simulink model "case5"  (R2024b)
settings: Solver=FixedStepAuto  StartTime=0  StopTime=1  FixedStep=1e-7  RelTol=1e-3
values from neighbouring files (symbols this model uses):
  SG_D_1_D = 0.01056    [IEEE9_case_parameters.m]    (also in case1_parameters.m; case2_parameters.m; case3_parameters.m; case4_parameters.m)
  SG_D_1_EnableSaturation = 0    [IEEE9_case_parameters.m]    (also in case1_parameters.m; case2_parameters.m; case3_parameters.m; case4_parameters.m)
  SG_D_1_f0 = 60    [IEEE9_case_parameters.m]    (also in case1_parameters.m; case2_parameters.m; case3_parameters.m; case4_parameters.m)
  SG_D_1_H = 7.5    [IEEE9_case_parameters.m]    (also in case1_parameters.m; case2_parameters.m; case3_parameters.m; case4_parameters.m)
  SG_D_1_K_A = 20    [IEEE9_case_parameters.m]    (also in case1_parameters.m; case2_parameters.m; case3_parameters.m; case4_parameters.m)
  SG_D_1_K_E = 1.000000e+1    (= 10)    [IEEE9_case_parameters.m]    (also in case1_parameters.m; case2_parameters.m; case3_parameters.m; case4_parameters.m)
  SG_D_1_K_F = 2.363    [IEEE9_case_parameters.m]    (also in case1_parameters.m; case2_parameters.m; case3_parameters.m; case4_parameters.m)
  SG_D_1_K_s = 0.5    [IEEE9_case_parameters.m]    (also in case1_parameters.m = 5; case2_parameters.m = 5; case3_parameters.m = 5; case4_parameters.m = 5)
  SG_D_1_R_a = 0.001088    [IEEE9_case_parameters.m]    (also in case1_parameters.m; case2_parameters.m; case3_parameters.m; case4_parameters.m)
  SG_D_1_S_A = 1    [IEEE9_case_parameters.m]    (also in case1_parameters.m; case2_parameters.m; case3_parameters.m; case4_parameters.m)
  SG_D_1_S_B = 0.103    [IEEE9_case_parameters.m]    (also in case1_parameters.m; case2_parameters.m; case3_parameters.m; case4_parameters.m)
  SG_D_1_S_N = 10.659857    [IEEE9_case_parameters.m]    (also in case1_parameters.m; case2_parameters.m; case3_parameters.m; case4_parameters.m)
  SG_D_1_SpeedPara = 200    [IEEE9_case_parameters.m]    (also in case1_parameters.m; case2_parameters.m; case3_parameters.m; case4_parameters.m)
  SG_D_1_T_0 = 0.720173    [IEEE9_case_parameters.m]    (also in case1_parameters.m = 0.755522; case2_parameters.m = 0.808931; case3_parameters.m = 0.869402; case4_parameters.m = 0.729316)
  SG_D_1_T_1 = 0.3    [IEEE9_case_parameters.m]    (also in case1_parameters.m; case2_parameters.m; case3_parameters.m; case4_parameters.m)
  SG_D_1_T_2 = 0.05    [IEEE9_case_parameters.m]    (also in case1_parameters.m; case2_parameters.m; case3_parameters.m; case4_parameters.m)
  SG_D_1_T_3 = 0.02    [IEEE9_case_parameters.m]    (also in case1_parameters.m; case2_parameters.m; case3_parameters.m; case4_parameters.m)
  SG_D_1_T_4 = 0.005    [IEEE9_case_parameters.m]    (also in case1_parameters.m; case2_parameters.m; case3_parameters.m; case4_parameters.m)
  SG_D_1_T_A = 0.02    [IEEE9_case_parameters.m]    (also in case1_parameters.m; case2_parameters.m; case3_parameters.m; case4_parameters.m)
  SG_D_1_T_dd = 8.000000e+0    (= 8)    [IEEE9_case_parameters.m]    (also in case1_parameters.m; case2_parameters.m; case3_parameters.m; case4_parameters.m)
  SG_D_1_T_ddd = 0.04    [IEEE9_case_parameters.m]    (also in case1_parameters.m; case2_parameters.m; case3_parameters.m; case4_parameters.m)
  SG_D_1_T_E = 0.314    [IEEE9_case_parameters.m]    (also in case1_parameters.m; case2_parameters.m; case3_parameters.m; case4_parameters.m)
  SG_D_1_T_F = 0.35    [IEEE9_case_parameters.m]    (also in case1_parameters.m; case2_parameters.m; case3_parameters.m; case4_parameters.m)
  SG_D_1_T_qd = 0.8    [IEEE9_case_parameters.m]    (also in case1_parameters.m; case2_parameters.m; case3_parameters.m; case4_parameters.m)
  SG_D_1_T_qdd = 0.02    [IEEE9_case_parameters.m]    (also in case1_parameters.m; case2_parameters.m; case3_parameters.m; case4_parameters.m)
  SG_D_1_T_speed = 0.1    [IEEE9_case_parameters.m]    (also in case1_parameters.m = 200; case2_parameters.m = 200; case3_parameters.m = 200; case4_parameters.m = 200)
  SG_D_1_T_w = 0.5    [IEEE9_case_parameters.m]    (also in case1_parameters.m; case2_parameters.m; case3_parameters.m; case4_parameters.m)
  SG_D_1_V_ref = 1.990276    [IEEE9_case_parameters.m]    (also in case1_parameters.m = 2.042296; case2_parameters.m = 2.051388; case3_parameters.m = 2.089584; case4_parameters.m = 2.01845)
  SG_D_1_w_ref = 376.991118    [IEEE9_case_parameters.m]    (also in case1_parameters.m; case2_parameters.m; case3_parameters.m; case4_parameters.m)
  SG_D_1_wb = 6.000000e+1    (= 60)    [IEEE9_case_parameters.m]    (also in case1_parameters.m; case2_parameters.m; case3_parameters.m; case4_parameters.m)
  SG_D_1_x_d = 1.9    [IEEE9_case_parameters.m]    (also in case1_parameters.m; case2_parameters.m; case3_parameters.m; case4_parameters.m)
  SG_D_1_x_dd = 0.302    [IEEE9_case_parameters.m]    (also in case1_parameters.m; case2_parameters.m; case3_parameters.m; case4_parameters.m)
  SG_D_1_x_ddd = 0.204    [IEEE9_case_parameters.m]    (also in case1_parameters.m; case2_parameters.m; case3_parameters.m; case4_parameters.m)
  SG_D_1_x_l = 0.05    [IEEE9_case_parameters.m]    (also in case1_parameters.m; case2_parameters.m; case3_parameters.m; case4_parameters.m)
  SG_D_1_x_q = 1.3    [IEEE9_case_parameters.m]    (also in case1_parameters.m; case2_parameters.m; case3_parameters.m; case4_parameters.m)
  SG_D_1_x_qd = 0.5    [IEEE9_case_parameters.m]    (also in case1_parameters.m; case2_parameters.m; case3_parameters.m; case4_parameters.m)
  SG_D_1_x_qdd = 0.3    [IEEE9_case_parameters.m]    (also in case1_parameters.m; case2_parameters.m; case3_parameters.m; case4_parameters.m)
  SG_D_2_D = 0.02    [IEEE9_case_parameters.m]    (also in case1_parameters.m; case2_parameters.m; case3_parameters.m; case4_parameters.m)
  SG_D_2_EnableSaturation = 0    [IEEE9_case_parameters.m]    (also in case1_parameters.m; case2_parameters.m; case3_parameters.m; case4_parameters.m)
  SG_D_2_f0 = 60    [IEEE9_case_parameters.m]    (also in case1_parameters.m; case2_parameters.m; case3_parameters.m; case4_parameters.m)
  SG_D_2_H = 8.000000e+0    (= 8)    [IEEE9_case_parameters.m]    (also in case1_parameters.m; case2_parameters.m; case3_parameters.m; case4_parameters.m)
  SG_D_2_K_A = 20    [IEEE9_case_parameters.m]    (also in case1_parameters.m; case2_parameters.m; case3_parameters.m; case4_parameters.m)
  SG_D_2_K_E = 1.000000e+1    (= 10)    [IEEE9_case_parameters.m]    (also in case1_parameters.m; case2_parameters.m; case3_parameters.m; case4_parameters.m)
  SG_D_2_K_F = 2.363    [IEEE9_case_parameters.m]    (also in case1_parameters.m; case2_parameters.m; case3_parameters.m; case4_parameters.m)
  SG_D_2_K_s = 0.5    [IEEE9_case_parameters.m]    (also in case1_parameters.m = 4; case2_parameters.m = 4; case3_parameters.m = 4; case4_parameters.m = 4)
  SG_D_2_R_a = 0.001088    [IEEE9_case_parameters.m]    (also in case1_parameters.m; case2_parameters.m; case3_parameters.m; case4_parameters.m)
  SG_D_2_S_A = 1    [IEEE9_case_parameters.m]    (also in case1_parameters.m; case2_parameters.m; case3_parameters.m; case4_parameters.m)
  SG_D_2_S_B = 0.103    [IEEE9_case_parameters.m]    (also in case1_parameters.m; case2_parameters.m; case3_parameters.m; case4_parameters.m)
  SG_D_2_S_N = 10.659857    [IEEE9_case_parameters.m]    (also in case1_parameters.m; case2_parameters.m; case3_parameters.m; case4_parameters.m)
  SG_D_2_SpeedPara = 200    [IEEE9_case_parameters.m]    (also in case1_parameters.m; case2_parameters.m; case3_parameters.m; case4_parameters.m)
  SG_D_2_T_0 = 1.632913    [IEEE9_case_parameters.m]    (also in case1_parameters.m = 1.632925; case2_parameters.m = 1.632915; case3_parameters.m = 1.632914; case4_parameters.m = 1.632927)
  SG_D_2_T_1 = 0.2    [IEEE9_case_parameters.m]    (also in case1_parameters.m; case2_parameters.m; case3_parameters.m; case4_parameters.m)
  SG_D_2_T_2 = 0.05    [IEEE9_case_parameters.m]    (also in case1_parameters.m; case2_parameters.m; case3_parameters.m; case4_parameters.m)
  SG_D_2_T_3 = 0.02    [IEEE9_case_parameters.m]    (also in case1_parameters.m; case2_parameters.m; case3_parameters.m; case4_parameters.m)
  SG_D_2_T_4 = 0.005    [IEEE9_case_parameters.m]    (also in case1_parameters.m; case2_parameters.m; case3_parameters.m; case4_parameters.m)
  SG_D_2_T_A = 0.02    [IEEE9_case_parameters.m]    (also in case1_parameters.m; case2_parameters.m; case3_parameters.m; case4_parameters.m)
  SG_D_2_T_dd = 7.9    [IEEE9_case_parameters.m]    (also in case1_parameters.m; case2_parameters.m; case3_parameters.m; case4_parameters.m)
  SG_D_2_T_ddd = 0.04    [IEEE9_case_parameters.m]    (also in case1_parameters.m; case2_parameters.m; case3_parameters.m; case4_parameters.m)
  SG_D_2_T_E = 0.314    [IEEE9_case_parameters.m]    (also in case1_parameters.m; case2_parameters.m; case3_parameters.m; case4_parameters.m)
  SG_D_2_T_F = 0.35    [IEEE9_case_parameters.m]    (also in case1_parameters.m; case2_parameters.m; case3_parameters.m; case4_parameters.m)
  SG_D_2_T_qd = 0.8    [IEEE9_case_parameters.m]    (also in case1_parameters.m; case2_parameters.m; case3_parameters.m; case4_parameters.m)
  SG_D_2_T_qdd = 0.015    [IEEE9_case_parameters.m]    (also in case1_parameters.m; case2_parameters.m; case3_parameters.m; case4_parameters.m)
  SG_D_2_T_speed = 0.1    [IEEE9_case_parameters.m]    (also in case1_parameters.m = 150; case2_parameters.m = 150; case3_parameters.m = 150; case4_parameters.m = 150)
  SG_D_2_T_w = 0.35    [IEEE9_case_parameters.m]    (also in case1_parameters.m; case2_parameters.m; case3_parameters.m; case4_parameters.m)
  SG_D_2_V_ref = 2.58547    [IEEE9_case_parameters.m]    (also in case1_parameters.m = 2.597896; case2_parameters.m = 2.587136; case3_parameters.m = 2.586042; case4_parameters.m = 2.599679)
  SG_D_2_w_ref = 376.991118    [IEEE9_case_parameters.m]    (also in case1_parameters.m; case2_parameters.m; case3_parameters.m; case4_parameters.m)
  SG_D_2_wb = 6.000000e+1    (= 60)    [IEEE9_case_parameters.m]    (also in case1_parameters.m; case2_parameters.m; case3_parameters.m; case4_parameters.m)
  SG_D_2_x_d = 1.8    [IEEE9_case_parameters.m]    (also in case1_parameters.m; case2_parameters.m; case3_parameters.m; case4_parameters.m)
  SG_D_2_x_dd = 0.302    [IEEE9_case_parameters.m]    (also in case1_parameters.m; case2_parameters.m; case3_parameters.m; case4_parameters.m)
  SG_D_2_x_ddd = 0.204    [IEEE9_case_parameters.m]    (also in case1_parameters.m; case2_parameters.m; case3_parameters.m; case4_parameters.m)
  SG_D_2_x_l = 0.05    [IEEE9_case_parameters.m]    (also in case1_parameters.m; case2_parameters.m; case3_parameters.m; case4_parameters.m)
  SG_D_2_x_q = 1.25    [IEEE9_case_parameters.m]    (also in case1_parameters.m; case2_parameters.m; case3_parameters.m; case4_parameters.m)
  SG_D_2_x_qd = 0.5    [IEEE9_case_parameters.m]    (also in case1_parameters.m; case2_parameters.m; case3_parameters.m; case4_parameters.m)
  SG_D_2_x_qdd = 0.3    [IEEE9_case_parameters.m]    (also in case1_parameters.m; case2_parameters.m; case3_parameters.m; case4_parameters.m)
  SG_D_3_D = 0.02    [IEEE9_case_parameters.m]    (also in case1_parameters.m; case2_parameters.m; case3_parameters.m; case4_parameters.m)
  SG_D_3_EnableSaturation = 0    [IEEE9_case_parameters.m]    (also in case1_parameters.m; case2_parameters.m; case3_parameters.m; case4_parameters.m)
  SG_D_3_f0 = 60    [IEEE9_case_parameters.m]    (also in case1_parameters.m; case2_parameters.m; case3_parameters.m; case4_parameters.m)
  SG_D_3_H = 7.7    [IEEE9_case_parameters.m]    (also in case1_parameters.m; case2_parameters.m; case3_parameters.m; case4_parameters.m)
  SG_D_3_K_A = 20    [IEEE9_case_parameters.m]    (also in case1_parameters.m; case2_parameters.m; case3_parameters.m; case4_parameters.m)
  SG_D_3_K_E = 1.000000e+1    (= 10)    [IEEE9_case_parameters.m]    (also in case1_parameters.m; case2_parameters.m; case3_parameters.m; case4_parameters.m)
  SG_D_3_K_F = 2.363    [IEEE9_case_parameters.m]    (also in case1_parameters.m; case2_parameters.m; case3_parameters.m; case4_parameters.m)
  SG_D_3_K_s = 0.2    [IEEE9_case_parameters.m]    (also in case1_parameters.m = 2; case2_parameters.m = 2; case3_parameters.m = 2; case4_parameters.m = 2)
  SG_D_3_R_a = 0.001088    [IEEE9_case_parameters.m]    (also in case1_parameters.m; case2_parameters.m; case3_parameters.m; case4_parameters.m)
  SG_D_3_S_A = 1    [IEEE9_case_parameters.m]    (also in case1_parameters.m; case2_parameters.m; case3_parameters.m; case4_parameters.m)
  SG_D_3_S_B = 0.103    [IEEE9_case_parameters.m]    (also in case1_parameters.m; case2_parameters.m; case3_parameters.m; case4_parameters.m)
  SG_D_3_S_N = 10.659857    [IEEE9_case_parameters.m]    (also in case1_parameters.m; case2_parameters.m; case3_parameters.m; case4_parameters.m)
  SG_D_3_SpeedPara = 200    [IEEE9_case_parameters.m]    (also in case1_parameters.m; case2_parameters.m; case3_parameters.m; case4_parameters.m)
  SG_D_3_T_0 = 0.850788    [IEEE9_case_parameters.m]    (also in case1_parameters.m = 0.850786; case2_parameters.m = 0.850787; case3_parameters.m; case4_parameters.m = 0.850786)
  SG_D_3_T_1 = 0.2    [IEEE9_case_parameters.m]    (also in case1_parameters.m; case2_parameters.m; case3_parameters.m; case4_parameters.m)
  SG_D_3_T_2 = 0.05    [IEEE9_case_parameters.m]    (also in case1_parameters.m; case2_parameters.m; case3_parameters.m; case4_parameters.m)
  SG_D_3_T_3 = 0.02    [IEEE9_case_parameters.m]    (also in case1_parameters.m; case2_parameters.m; case3_parameters.m; case4_parameters.m)
  SG_D_3_T_4 = 0.005    [IEEE9_case_parameters.m]    (also in case1_parameters.m; case2_parameters.m; case3_parameters.m; case4_parameters.m)
  SG_D_3_T_A = 0.02    [IEEE9_case_parameters.m]    (also in case1_parameters.m; case2_parameters.m; case3_parameters.m; case4_parameters.m)
  SG_D_3_T_dd = 8.1    [IEEE9_case_parameters.m]    (also in case1_parameters.m; case2_parameters.m; case3_parameters.m; case4_parameters.m)
  SG_D_3_T_ddd = 0.04    [IEEE9_case_parameters.m]    (also in case1_parameters.m; case2_parameters.m; case3_parameters.m; case4_parameters.m)
  SG_D_3_T_E = 0.314    [IEEE9_case_parameters.m]    (also in case1_parameters.m; case2_parameters.m; case3_parameters.m; case4_parameters.m)
  SG_D_3_T_F = 0.35    [IEEE9_case_parameters.m]    (also in case1_parameters.m; case2_parameters.m; case3_parameters.m; case4_parameters.m)
  SG_D_3_T_qd = 0.8    [IEEE9_case_parameters.m]    (also in case1_parameters.m; case2_parameters.m; case3_parameters.m; case4_parameters.m)
  SG_D_3_T_qdd = 0.015    [IEEE9_case_parameters.m]    (also in case1_parameters.m; case2_parameters.m; case3_parameters.m; case4_parameters.m)
  SG_D_3_T_speed = 0.1    [IEEE9_case_parameters.m]    (also in case1_parameters.m = 180; case2_parameters.m = 180; case3_parameters.m = 180; case4_parameters.m = 180)
  SG_D_3_T_w = 0.4    [IEEE9_case_parameters.m]    (also in case1_parameters.m; case2_parameters.m; case3_parameters.m; case4_parameters.m)
  SG_D_3_V_ref = 1.892727    [IEEE9_case_parameters.m]    (also in case1_parameters.m = 1.906439; case2_parameters.m = 1.895535; case3_parameters.m = 1.892105; case4_parameters.m = 1.906598)
  SG_D_3_w_ref = 376.991118    [IEEE9_case_parameters.m]    (also in case1_parameters.m; case2_parameters.m; case3_parameters.m; case4_parameters.m)
  SG_D_3_wb = 6.000000e+1    (= 60)    [IEEE9_case_parameters.m]    (also in case1_parameters.m; case2_parameters.m; case3_parameters.m; case4_parameters.m)
  SG_D_3_x_d = 1.85    [IEEE9_case_parameters.m]    (also in case1_parameters.m; case2_parameters.m; case3_parameters.m; case4_parameters.m)
  SG_D_3_x_dd = 0.302    [IEEE9_case_parameters.m]    (also in case1_parameters.m; case2_parameters.m; case3_parameters.m; case4_parameters.m)
  SG_D_3_x_ddd = 0.204    [IEEE9_case_parameters.m]    (also in case1_parameters.m; case2_parameters.m; case3_parameters.m; case4_parameters.m)
  SG_D_3_x_l = 0.05    [IEEE9_case_parameters.m]    (also in case1_parameters.m; case2_parameters.m; case3_parameters.m; case4_parameters.m)
  SG_D_3_x_q = 1.2    [IEEE9_case_parameters.m]    (also in case1_parameters.m; case2_parameters.m; case3_parameters.m; case4_parameters.m)
  SG_D_3_x_qd = 0.5    [IEEE9_case_parameters.m]    (also in case1_parameters.m; case2_parameters.m; case3_parameters.m; case4_parameters.m)
  SG_D_3_x_qdd = 0.3    [IEEE9_case_parameters.m]    (also in case1_parameters.m; case2_parameters.m; case3_parameters.m; case4_parameters.m)
(part 11 of 12)

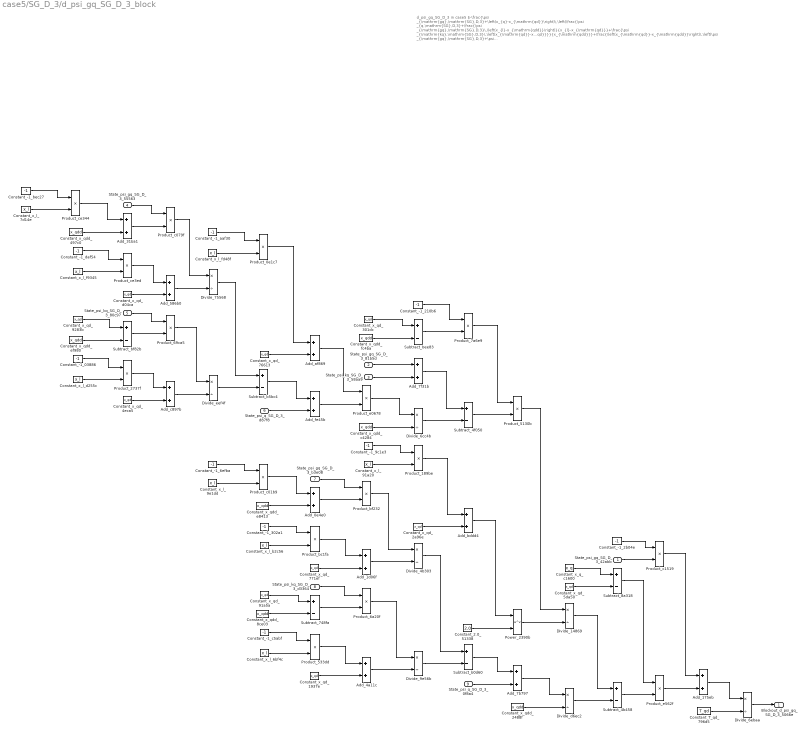
== system case5/SG_D_3/d_psi_gq_SG_D_3_block ==
  note: d_psi_gq_SG_D_3 in case5
      | $-\frac{\psi _{\mathrm{gq},\mathrm{SG},D,3}+\left(x_{q}-x_{\mathrm{qd}}\right)\,\left(\frac{\psi _{q,\mathrm{SG},D,3}+\frac{\psi _{\mathrm{gq},\mathrm{SG},D,3}\,\left(x_{l}-x_{\mathrm{qdd}}\right)}{x_{l}-x_{\mathrm{qd}}}+\frac{\psi _{\mathrm{kq},\mathrm{SG},D,3}\,\left(x_{\mathrm{qd}}-x_{\mathrm{qdd}}\right)}{x_{l}-x_{\mathrm{qd}}}}{x_{\mathrm{qdd}}}+\frac{\left(x_{\mathrm{qd}}-x_{\mathrm{qdd}}\right)\,\left(\psi _{\mathrm{gq},\mathrm{SG},D,3}+\psi _{\mathrm{kq},\mathrm{SG},D,3}+\frac{\left(x_{l}-x_{\mathrm{qd}}\right)\,\left(\psi _{q,\mathrm{SG},D,3}+\frac{\psi _{\mathrm{gq},\mathrm{SG},D,3}\,\left(x_{l}-x_{\mathrm{qdd}}\right)}{x_{l}-x_{\mathrm{qd}}}+\frac{\psi _{\mathrm{kq},\mathrm{SG},D,3}\,\left(x_{\mathrm{qd}}-x_{\mathrm{qdd}}\right)}{x_{l}-x_{\mathrm{qd}}}\right)}{x_{\mathrm{qdd}}}\right)}{{\left(x_{l}-x_{\mathrm{qd}}\right)}^2}\right)}{T_{\mathrm{qd}}}$
      | Automatically generated on 2025-10-31 19:12:39 .
  State_psi_gq_SG_D_3_42abb : Inport
  State_psi_gq_SG_D_3_81b5d : Inport  Port=2
  State_psi_kq_SG_D_3_58aa9 : Inport  Port=3
  State_psi_gq_SG_D_3_55563 : Inport  Port=4
  State_psi_kq_SG_D_3_80c97 : Inport  Port=5
  State_psi_q_SG_D_3_d87f8 : Inport  Port=6
  State_psi_gq_SG_D_3_b3e08 : Inport  Port=7
  State_psi_kq_SG_D_3_d3364 : Inport  Port=8
  State_psi_q_SG_D_3_0f8a4 : Inport  Port=9
  Add_0e4e0 : Sum
  Add_175eb : Sum
  Add_1d06f : Sum
  Add_31ba1 : Sum
  Add_4a11c : Sum
  Add_586b0 : Sum
  Add_7b797 : Sum
  Add_7f31b : Sum
  Add_af869 : Sum
  Add_bddd4 : Sum
  Add_c897b : Sum
  Add_fe45b : Sum
  Constant_-1_03886 : Constant  Value=-1
  Constant_-1_210b6 : Constant  Value=-1
  Constant_-1_2b04e : Constant  Value=-1
  Constant_-1_302a1 : Constant  Value=-1
  Constant_-1_6efba : Constant  Value=-1
  Constant_-1_9c1e3 : Constant  Value=-1
  Constant_-1_aaf30 : Constant  Value=-1
  Constant_-1_bec27 : Constant  Value=-1
  Constant_-1_c5abf : Constant  Value=-1
  Constant_-1_daf54 : Constant  Value=-1
  Constant_2.0_51338 : Constant  Value=2.0
  Constant_T_qd_796d5 : Constant  Value=T_qd
  Constant_x_l_6bf4c : Constant  Value=x_l
  Constant_x_l_7d14e : Constant  Value=x_l
  Constant_x_l_91a20 : Constant  Value=x_l
  Constant_x_l_9e1dd : Constant  Value=x_l
  Constant_x_l_b2c56 : Constant  Value=x_l
  Constant_x_l_d255c : Constant  Value=x_l
  Constant_x_l_f9345 : Constant  Value=x_l
  Constant_x_l_fd48f : Constant  Value=x_l
  Constant_x_q_c1600 : Constant  Value=x_q
  Constant_x_qd_1937e : Constant  Value=x_qd
  Constant_x_qd_2a96e : Constant  Value=x_qd
  Constant_x_qd_301dc : Constant  Value=x_qd
  Constant_x_qd_4eca5 : Constant  Value=x_qd
  Constant_x_qd_5da50 : Constant  Value=x_qd
  Constant_x_qd_76613 : Constant  Value=x_qd
  Constant_x_qd_771ef : Constant  Value=x_qd
  Constant_x_qd_91a5a : Constant  Value=x_qd
  Constant_x_qd_9283b : Constant  Value=x_qd
  Constant_x_qd_d04ca : Constant  Value=x_qd
  Constant_x_qdd_2488f : Constant  Value=x_qdd
  Constant_x_qdd_497c0 : Constant  Value=x_qdd
  Constant_x_qdd_8ce03 : Constant  Value=x_qdd
  Constant_x_qdd_c4284 : Constant  Value=x_qdd
  Constant_x_qdd_e8413 : Constant  Value=x_qdd
  Constant_x_qdd_ef980 : Constant  Value=x_qdd
  Constant_x_qdd_fc4ba : Constant  Value=x_qdd
  Divide_14869 : Product  Inputs=*/
  Divide_4b303 : Product  Inputs=*/
  Divide_6cc4b : Product  Inputs=*/
  Divide_6ebaa : Product  Inputs=*/
  Divide_75568 : Product  Inputs=*/
  Divide_9e56b : Product  Inputs=*/
  Divide_d6ec2 : Product  Inputs=*/
  Divide_eef4f : Product  Inputs=*/
  Power_2390b : Math  Operator=pow
  Product_0e1c7 : Product
  Product_189be : Product
  Product_2737f : Product
  Product_5130b : Product
  Product_533dd : Product
  Product_69ca5 : Product
  Product_6a20f : Product
  Product_7a6e9 : Product
  Product_bc1fa : Product
  Product_bf232 : Product
  Product_c01b9 : Product
  Product_c079f : Product
  Product_c1519 : Product
  Product_ce344 : Product
  Product_ce3ed : Product
  Product_e0678 : Product
  Product_e562f : Product
  Subtract_4b458 : Sum  Inputs=+-
  Subtract_4f050 : Sum  Inputs=+-
  Subtract_748fa : Sum  Inputs=+-
  Subtract_8a318 : Sum  Inputs=+-
  Subtract_b0d60 : Sum  Inputs=+-
  Subtract_b5bc4 : Sum  Inputs=+-
  Subtract_bee83 : Sum  Inputs=+-
  Subtract_bf82b : Sum  Inputs=+-
  Blockout_d_psi_gq_SG_D_3_5066e : Outport
  wires:
  Constant_x_l_91a20/1 -> Product_189be/2
  Constant_x_qd_9283b/1 -> Subtract_bf82b/1
  Add_af869/1 -> Product_e0678/1
  Constant_-1_bec27/1 -> Product_ce344/1
  Add_31ba1/1 -> Product_c079f/2
  Constant_x_qdd_ef980/1 -> Subtract_bf82b/2
  Constant_x_qd_76613/1 -> Add_af869/2
  Constant_x_l_7d14e/1 -> Product_ce344/2
  Constant_x_l_f9345/1 -> Product_ce3ed/2
  Add_4a11c/1 -> Divide_9e56b/2
  State_psi_kq_SG_D_3_58aa9/1 -> Add_7f31b/2
  Constant_x_qdd_497c0/1 -> Add_31ba1/2
  Product_ce344/1 -> Add_31ba1/1
  Constant_x_qd_1937e/1 -> Add_4a11c/2
  Product_7a6e9/1 -> Product_5130b/1
  Constant_-1_6efba/1 -> Product_c01b9/1
  Constant_-1_daf54/1 -> Product_ce3ed/1
  Constant_-1_03886/1 -> Product_2737f/1
  Constant_x_l_d255c/1 -> Product_2737f/2
  Constant_-1_210b6/1 -> Product_7a6e9/1
  Constant_-1_2b04e/1 -> Product_c1519/1
  State_psi_gq_SG_D_3_55563/1 -> Product_c079f/1
  Product_c01b9/1 -> Add_0e4e0/1
  Product_ce3ed/1 -> Add_586b0/1
  Product_533dd/1 -> Add_4a11c/1
  Constant_x_qd_d04ca/1 -> Add_586b0/2
  Constant_-1_302a1/1 -> Product_bc1fa/1
  State_psi_kq_SG_D_3_80c97/1 -> Product_69ca5/1
  Subtract_bf82b/1 -> Product_69ca5/2
  Product_2737f/1 -> Add_c897b/1
  Add_0e4e0/1 -> Product_bf232/2
  Add_586b0/1 -> Divide_75568/2
  Constant_x_qd_4eca5/1 -> Add_c897b/2
  Product_c079f/1 -> Divide_75568/1
  Constant_T_qd_796d5/1 -> Divide_6ebaa/2
  Product_bc1fa/1 -> Add_1d06f/1
  Product_69ca5/1 -> Divide_eef4f/1
  Product_6a20f/1 -> Divide_9e56b/1
  Add_c897b/1 -> Divide_eef4f/2
  Constant_-1_aaf30/1 -> Product_0e1c7/1
  Constant_x_qdd_c4284/1 -> Divide_6cc4b/2
  Constant_x_l_fd48f/1 -> Product_0e1c7/2
  Divide_75568/1 -> Subtract_b5bc4/1
  Constant_x_qd_5da50/1 -> Subtract_8a318/2
  Add_1d06f/1 -> Divide_4b303/2
  Divide_eef4f/1 -> Subtract_b5bc4/2
  Constant_x_l_9e1dd/1 -> Product_c01b9/2
  Product_0e1c7/1 -> Add_af869/1
  Constant_-1_9c1e3/1 -> Product_189be/1
  Constant_x_l_b2c56/1 -> Product_bc1fa/2
  Subtract_b5bc4/1 -> Add_fe45b/1
  State_psi_q_SG_D_3_d87f8/1 -> Add_fe45b/2
  Constant_-1_c5abf/1 -> Product_533dd/1
  Constant_x_qdd_e8413/1 -> Add_0e4e0/2
  Constant_x_qd_91a5a/1 -> Subtract_748fa/1
  Constant_x_qdd_8ce03/1 -> Subtract_748fa/2
  Constant_x_l_6bf4c/1 -> Product_533dd/2
  Add_fe45b/1 -> Product_e0678/2
  Constant_x_qdd_fc4ba/1 -> Subtract_bee83/2
  State_psi_gq_SG_D_3_b3e08/1 -> Product_bf232/1
  Constant_x_qd_771ef/1 -> Add_1d06f/2
  Divide_14869/1 -> Subtract_4b458/1
  State_psi_kq_SG_D_3_d3364/1 -> Product_6a20f/1
  Subtract_748fa/1 -> Product_6a20f/2
  Constant_x_qd_301dc/1 -> Subtract_bee83/1
  State_psi_gq_SG_D_3_81b5d/1 -> Add_7f31b/1
  Product_e0678/1 -> Divide_6cc4b/1
  Product_bf232/1 -> Divide_4b303/1
  Subtract_bee83/1 -> Product_7a6e9/2
  Add_7f31b/1 -> Subtract_4f050/1
  Divide_6cc4b/1 -> Subtract_4f050/2
  Product_189be/1 -> Add_bddd4/1
  Constant_x_qd_2a96e/1 -> Add_bddd4/2
  Divide_4b303/1 -> Subtract_b0d60/1
  Divide_9e56b/1 -> Subtract_b0d60/2
  Subtract_4f050/1 -> Product_5130b/2
  Add_bddd4/1 -> Power_2390b/1
  Constant_2.0_51338/1 -> Power_2390b/2
  Subtract_b0d60/1 -> Add_7b797/1
  State_psi_q_SG_D_3_0f8a4/1 -> Add_7b797/2
  Product_5130b/1 -> Divide_14869/1
  Power_2390b/1 -> Divide_14869/2
  Add_7b797/1 -> Divide_d6ec2/1
  Constant_x_qdd_2488f/1 -> Divide_d6ec2/2
  Constant_x_q_c1600/1 -> Subtract_8a318/1
  Divide_d6ec2/1 -> Subtract_4b458/2
  State_psi_gq_SG_D_3_42abb/1 -> Product_c1519/2
  Subtract_8a318/1 -> Product_e562f/1
  Subtract_4b458/1 -> Product_e562f/2
  Product_c1519/1 -> Add_175eb/1
  Product_e562f/1 -> Add_175eb/2
  Add_175eb/1 -> Divide_6ebaa/1
  Divide_6ebaa/1 -> Blockout_d_psi_gq_SG_D_3_5066e/1

== system case5/SG_D_3/d_psi_kq_SG_D_3_block ==
  note: d_psi_kq_SG_D_3 in case5
      | $-\frac{\psi _{\mathrm{gq},\mathrm{SG},D,3}+\psi _{\mathrm{kq},\mathrm{SG},D,3}+\frac{\left(x_{l}-x_{\mathrm{qd}}\right)\,\left(\psi _{q,\mathrm{SG},D,3}+\frac{\psi _{\mathrm{gq},\mathrm{SG},D,3}\,\left(x_{l}-x_{\mathrm{qdd}}\right)}{x_{l}-x_{\mathrm{qd}}}+\frac{\psi _{\mathrm{kq},\mathrm{SG},D,3}\,\left(x_{\mathrm{qd}}-x_{\mathrm{qdd}}\right)}{x_{l}-x_{\mathrm{qd}}}\right)}{x_{\mathrm{qdd}}}}{T_{\mathrm{qdd}}}$
      | Automatically generated on 2025-10-31 19:12:43 .
  State_psi_gq_SG_D_3_4cb6a : Inport
  State_psi_kq_SG_D_3_1fc99 : Inport  Port=2
  State_psi_gq_SG_D_3_b2b08 : Inport  Port=3
  State_psi_kq_SG_D_3_7e333 : Inport  Port=4
  State_psi_q_SG_D_3_1522f : Inport  Port=5
  Add_42471 : Sum
  Add_97b8c : Sum
  Add_980fe : Sum
  Add_ac8f7 : Sum
  Add_b61cb : Sum
  Add_f607d : Sum
  Constant_-1_8b77c : Constant  Value=-1
  Constant_-1_9ca42 : Constant  Value=-1
  Constant_-1_d760d : Constant  Value=-1
  Constant_-1_d8fd2 : Constant  Value=-1
  Constant_-1_f8a23 : Constant  Value=-1
  Constant_T_qdd_3f294 : Constant  Value=T_qdd
  Constant_x_l_2ca16 : Constant  Value=x_l
  Constant_x_l_7a469 : Constant  Value=x_l
  Constant_x_l_98c4a : Constant  Value=x_l
  Constant_x_l_df7a3 : Constant  Value=x_l
  Constant_x_qd_662a6 : Constant  Value=x_qd
  Constant_x_qd_e69a7 : Constant  Value=x_qd
  Constant_x_qd_eee3f : Constant  Value=x_qd
  Constant_x_qd_fb7dc : Constant  Value=x_qd
  Constant_x_qdd_2435d : Constant  Value=x_qdd
  Constant_x_qdd_6703f : Constant  Value=x_qdd
  Constant_x_qdd_dc427 : Constant  Value=x_qdd
  Divide_33b3b : Product  Inputs=*/
  Divide_90e6d : Product  Inputs=*/
  Divide_baf14 : Product  Inputs=*/
  Divide_c9465 : Product  Inputs=*/
  Product_09bed : Product
  Product_0a072 : Product
  Product_0f95d : Product
  Product_17894 : Product
  Product_3a07f : Product
  Product_79449 : Product
  Product_93ee1 : Product
  Product_b3933 : Product
  Subtract_7b4c8 : Sum  Inputs=+-
  Subtract_84736 : Sum  Inputs=+-
  Subtract_d86bb : Sum  Inputs=+-
  Blockout_d_psi_kq_SG_D_3_acb7b : Outport
  wires:
  State_psi_q_SG_D_3_1522f/1 -> Add_b61cb/2
  Constant_-1_8b77c/1 -> Product_79449/1
  Constant_-1_d8fd2/1 -> Product_b3933/1
  Constant_-1_d760d/1 -> Product_93ee1/1
  Constant_x_l_7a469/1 -> Product_79449/2
  Constant_x_qdd_6703f/1 -> Add_980fe/2
  Product_0f95d/1 -> Add_97b8c/1
  Constant_x_l_2ca16/1 -> Product_b3933/2
  Constant_x_qd_e69a7/1 -> Subtract_84736/1
  Product_b3933/1 -> Add_980fe/1
  Constant_x_l_98c4a/1 -> Product_0a072/2
  Constant_x_qdd_dc427/1 -> Subtract_84736/2
  Constant_-1_f8a23/1 -> Product_0f95d/1
  Constant_x_l_df7a3/1 -> Product_0f95d/2
  State_psi_gq_SG_D_3_b2b08/1 -> Product_09bed/1
  Add_980fe/1 -> Product_09bed/2
  Add_b61cb/1 -> Product_3a07f/2
  Product_79449/1 -> Add_42471/1
  Constant_x_qd_fb7dc/1 -> Add_42471/2
  State_psi_kq_SG_D_3_7e333/1 -> Product_17894/1
  Subtract_84736/1 -> Product_17894/2
  Add_42471/1 -> Divide_baf14/2
  Constant_x_qd_eee3f/1 -> Add_97b8c/2
  Product_09bed/1 -> Divide_baf14/1
  Product_17894/1 -> Divide_c9465/1
  Add_97b8c/1 -> Divide_c9465/2
  Constant_-1_9ca42/1 -> Product_0a072/1
  Divide_baf14/1 -> Subtract_7b4c8/1
  Add_f607d/1 -> Divide_90e6d/1
  Divide_c9465/1 -> Subtract_7b4c8/2
  Divide_90e6d/1 -> Blockout_d_psi_kq_SG_D_3_acb7b/1
  Product_0a072/1 -> Add_ac8f7/1
  Constant_x_qd_662a6/1 -> Add_ac8f7/2
  Subtract_7b4c8/1 -> Add_b61cb/1
  State_psi_gq_SG_D_3_4cb6a/1 -> Product_93ee1/2
  Add_ac8f7/1 -> Product_3a07f/1
  Constant_T_qdd_3f294/1 -> Divide_90e6d/2
  Product_93ee1/1 -> Subtract_d86bb/1
  State_psi_kq_SG_D_3_1fc99/1 -> Subtract_d86bb/2
  Product_3a07f/1 -> Divide_33b3b/1
  Constant_x_qdd_2435d/1 -> Divide_33b3b/2
  Subtract_d86bb/1 -> Add_f607d/1
  Divide_33b3b/1 -> Add_f607d/2

== system case5/SG_D_3/d_psi_q_SG_D_3_block ==
  note: d_psi_q_SG_D_3 in case5
      | $2\,\pi \,f_{0}\,\left(v_{d,\mathrm{SG},D,3}\,\cos\left(\theta _{\mathrm{SG},D,3}\right)+v_{q,\mathrm{SG},D,3}\,\sin\left(\theta _{\mathrm{SG},D,3}\right)-\frac{R_{a}\,\left(\psi _{q,\mathrm{SG},D,3}+\frac{\psi _{\mathrm{gq},\mathrm{SG},D,3}\,\left(x_{l}-x_{\mathrm{qdd}}\right)}{x_{l}-x_{\mathrm{qd}}}+\frac{\psi _{\mathrm{kq},\mathrm{SG},D,3}\,\left(x_{\mathrm{qd}}-x_{\mathrm{qdd}}\right)}{x_{l}-x_{\mathrm{qd}}}\right)}{x_{\mathrm{qdd}}}-\frac{\psi _{d,\mathrm{SG},D,3}\,w_{\mathrm{SG},D,3}}{2\,f_{0}\,\pi }\right)$
      | Automatically generated on 2025-10-31 19:12:21 .
  State_psi_gq_SG_D_3_1dddd : Inport
  State_psi_kq_SG_D_3_924ec : Inport  Port=2
  State_psi_q_SG_D_3_33284 : Inport  Port=3
  Input_v_d_SG_D_3_84d49 : Inport  Port=4
  State_theta_SG_D_3_74150 : Inport  Port=5
  Input_v_q_SG_D_3_69553 : Inport  Port=6
  State_theta_SG_D_3_ee4f0 : Inport  Port=7
  State_psi_d_SG_D_3_b8185 : Inport  Port=8
  State_w_SG_D_3_7587a : Inport  Port=9
  Add_0135e : Sum
  Add_6da62 : Sum
  Add_e06d9 : Sum
  Add_e2e1a : Sum
  Add_f1ad9 : Sum
  Constant_-1_3a3c9 : Constant  Value=-1
  Constant_-1_9aa02 : Constant  Value=-1
  Constant_-1_a4dec : Constant  Value=-1
  Constant_-2.0_cd1ed : Constant  Value=-2.0
  Constant_2.0_e0a03 : Constant  Value=2.0
  Constant_R_a_2b4eb : Constant  Value=R_a
  Constant_f0_a886c : Constant  Value=f0
  Constant_f0_e42f2 : Constant  Value=f0
  Constant_pi_2a66a : Constant  Value=pi
  Constant_pi_b7ce5 : Constant  Value=pi
  Constant_x_l_38c93 : Constant  Value=x_l
  Constant_x_l_95186 : Constant  Value=x_l
  Constant_x_l_96a9a : Constant  Value=x_l
  Constant_x_qd_518f3 : Constant  Value=x_qd
  Constant_x_qd_76935 : Constant  Value=x_qd
  Constant_x_qd_be2b6 : Constant  Value=x_qd
  Constant_x_qdd_72bab : Constant  Value=x_qdd
  Constant_x_qdd_79a63 : Constant  Value=x_qdd
  Constant_x_qdd_88577 : Constant  Value=x_qdd
  Divide_69726 : Product  Inputs=*/
  Divide_6bb03 : Product  Inputs=*/
  Divide_85693 : Product  Inputs=*/
  Divide_cacec : Product  Inputs=*/
  MathFunc_cos_15b0f : Trigonometry  Operator=cos
  MathFunc_sin_5f384 : Trigonometry
  Product_029c0 : Product
  Product_193b5 : Product
  Product_1a6f5 : Product
  Product_3225c : Product
  Product_338b4 : Product
  Product_3f55e : Product
  Product_4baa4 : Product
  Product_54bdc : Product
  Product_732e6 : Product
  Product_9dcf3 : Product
  Product_a185d : Product
  Product_c6890 : Product
  Product_d2c1e : Product
  Product_f2d8f : Product
  Subtract_0dfba : Sum  Inputs=+-
  Subtract_20ea1 : Sum  Inputs=+-
  Subtract_a2acb : Sum  Inputs=+-
  Subtract_f404d : Sum  Inputs=+-
  Blockout_d_psi_q_SG_D_3_a4a1c : Outport
  wires:
  Constant_x_qd_76935/1 -> Subtract_20ea1/1
  Constant_pi_2a66a/1 -> Product_c6890/2
  Product_d2c1e/1 -> Divide_cacec/1
  Constant_x_l_96a9a/1 -> Product_f2d8f/2
  Constant_f0_a886c/1 -> Product_3f55e/2
  State_w_SG_D_3_7587a/1 -> Product_193b5/2
  Constant_-1_a4dec/1 -> Product_a185d/1
  Constant_x_qdd_72bab/1 -> Add_6da62/2
  Input_v_d_SG_D_3_84d49/1 -> Product_1a6f5/1
  Constant_x_qdd_79a63/1 -> Subtract_20ea1/2
  Constant_x_l_38c93/1 -> Product_a185d/2
  Divide_6bb03/1 -> Add_e2e1a/2
  Product_a185d/1 -> Add_6da62/1
  Constant_2.0_e0a03/1 -> Product_c6890/1
  Add_f1ad9/1 -> Product_d2c1e/2
  Constant_-1_3a3c9/1 -> Product_f2d8f/1
  Constant_x_qd_518f3/1 -> Add_e06d9/2
  Constant_-1_9aa02/1 -> Product_732e6/1
  Subtract_a2acb/1 -> Subtract_0dfba/1
  Constant_x_l_95186/1 -> Product_732e6/2
  Subtract_0dfba/1 -> Add_e2e1a/1
  Constant_f0_e42f2/1 -> Product_3225c/2
  State_theta_SG_D_3_ee4f0/1 -> MathFunc_sin_5f384/1
  Constant_x_qd_be2b6/1 -> Add_0135e/2
  State_psi_gq_SG_D_3_1dddd/1 -> Product_9dcf3/1
  Add_6da62/1 -> Product_9dcf3/2
  Product_c6890/1 -> Product_3225c/1
  Product_f2d8f/1 -> Add_0135e/1
  State_psi_kq_SG_D_3_924ec/1 -> Product_54bdc/1
  Subtract_20ea1/1 -> Product_54bdc/2
  Product_732e6/1 -> Add_e06d9/1
  MathFunc_sin_5f384/1 -> Product_338b4/2
  Product_9dcf3/1 -> Divide_69726/1
  Product_3225c/1 -> Divide_6bb03/2
  Add_0135e/1 -> Divide_69726/2
  Product_54bdc/1 -> Divide_85693/1
  Add_e06d9/1 -> Divide_85693/2
  Input_v_q_SG_D_3_69553/1 -> Product_338b4/1
  Divide_69726/1 -> Subtract_f404d/1
  Subtract_f404d/1 -> Add_f1ad9/1
  Divide_85693/1 -> Subtract_f404d/2
  Divide_cacec/1 -> Subtract_a2acb/1
  State_psi_q_SG_D_3_33284/1 -> Add_f1ad9/2
  Product_338b4/1 -> Subtract_0dfba/2
  Constant_R_a_2b4eb/1 -> Product_d2c1e/1
  State_theta_SG_D_3_74150/1 -> MathFunc_cos_15b0f/1
  Constant_x_qdd_88577/1 -> Divide_cacec/2
  MathFunc_cos_15b0f/1 -> Product_1a6f5/2
  Constant_-2.0_cd1ed/1 -> Product_4baa4/1
  Product_1a6f5/1 -> Subtract_a2acb/2
  State_psi_d_SG_D_3_b8185/1 -> Product_193b5/1
  Constant_pi_b7ce5/1 -> Product_4baa4/2
  Product_193b5/1 -> Divide_6bb03/1
  Product_4baa4/1 -> Product_3f55e/1
  Product_3f55e/1 -> Product_029c0/1
  Add_e2e1a/1 -> Product_029c0/2
  Product_029c0/1 -> Blockout_d_psi_q_SG_D_3_a4a1c/1

== system case5/SG_D_3/d_theta_SG_D_3_block ==
  note: d_theta_SG_D_3 in case5
      | $w_{\mathrm{SG},D,3}-2\,\pi \,f_{0}$
      | Automatically generated on 2025-10-31 19:12:50 .
  State_w_SG_D_3_3c4ab : Inport
  Add_740f8 : Sum
  Constant_-2.0_dd5d4 : Constant  Value=-2.0
  Constant_f0_25804 : Constant  Value=f0
  Constant_pi_a3a68 : Constant  Value=pi
  Product_064f8 : Product
  Product_555fc : Product
  Blockout_d_theta_SG_D_3_6d326 : Outport
  wires:
  Constant_-2.0_dd5d4/1 -> Product_555fc/1
  Constant_pi_a3a68/1 -> Product_555fc/2
  State_w_SG_D_3_3c4ab/1 -> Add_740f8/2
  Product_555fc/1 -> Product_064f8/1
  Constant_f0_25804/1 -> Product_064f8/2
  Product_064f8/1 -> Add_740f8/1
  Add_740f8/1 -> Blockout_d_theta_SG_D_3_6d326/1

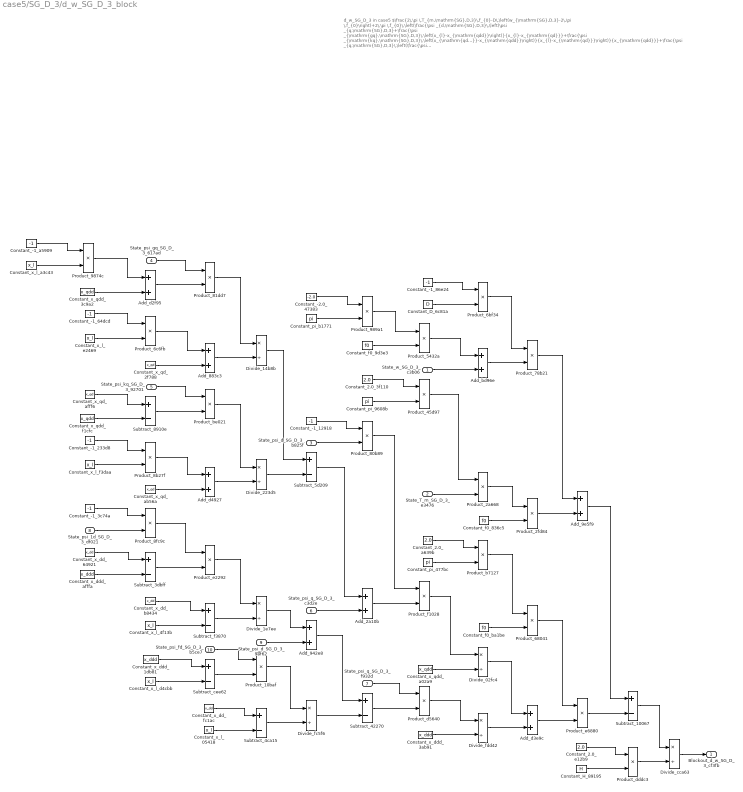
== system case5/SG_D_3/d_w_SG_D_3_block ==
  note: d_w_SG_D_3 in case5
      | $\frac{2\,\pi \,T_{m,\mathrm{SG},D,3}\,f_{0}-D\,\left(w_{\mathrm{SG},D,3}-2\,\pi \,f_{0}\right)+2\,\pi \,f_{0}\,\left(\frac{\psi _{d,\mathrm{SG},D,3}\,\left(\psi _{q,\mathrm{SG},D,3}+\frac{\psi _{\mathrm{gq},\mathrm{SG},D,3}\,\left(x_{l}-x_{\mathrm{qdd}}\right)}{x_{l}-x_{\mathrm{qd}}}+\frac{\psi _{\mathrm{kq},\mathrm{SG},D,3}\,\left(x_{\mathrm{qd}}-x_{\mathrm{qdd}}\right)}{x_{l}-x_{\mathrm{qd}}}\right)}{x_{\mathrm{qdd}}}+\frac{\psi _{q,\mathrm{SG},D,3}\,\left(\frac{\psi _{\mathrm{1d},\mathrm{SG},D,3}\,\left(x_{\mathrm{dd}}-x_{\mathrm{ddd}}\right)}{x_{\mathrm{dd}}-x_{l}}-\psi _{d,\mathrm{SG},D,3}+\frac{\psi _{\mathrm{fd},\mathrm{SG},D,3}\,\left(x_{\mathrm{ddd}}-x_{l}\right)}{x_{\mathrm{dd}}-x_{l}}\right)}{x_{\mathrm{ddd}}}\right)}{2\,H}$
      | Automatically generated on 2025-10-31 19:12:48 .
  State_w_SG_D_3_c3b06 : Inport
  State_T_m_SG_D_3_e3476 : Inport  Port=2
  State_psi_d_SG_D_3_b825f : Inport  Port=3
  State_psi_gq_SG_D_3_617ad : Inport  Port=4
  State_psi_kq_SG_D_3_92701 : Inport  Port=5
  State_psi_q_SG_D_3_c3d2e : Inport  Port=6
  State_psi_q_SG_D_3_f932d : Inport  Port=7
  State_psi_1d_SG_D_3_df021 : Inport  Port=8
  State_psi_d_SG_D_3_9af62 : Inport  Port=9
  State_psi_fd_SG_D_3_b5ce7 : Inport  Port=10
  Add_2a10b : Sum
  Add_883c3 : Sum
  Add_942e8 : Sum
  Add_9e5f9 : Sum
  Add_bd96e : Sum
  Add_d2f95 : Sum
  Add_d3e9c : Sum
  Add_d4927 : Sum
  Constant_-1_12918 : Constant  Value=-1
  Constant_-1_233d8 : Constant  Value=-1
  Constant_-1_3c74a : Constant  Value=-1
  Constant_-1_64dcd : Constant  Value=-1
  Constant_-1_86e24 : Constant  Value=-1
  Constant_-1_a5909 : Constant  Value=-1
  Constant_-2.0_47383 : Constant  Value=-2.0
  Constant_2.0_3f110 : Constant  Value=2.0
  Constant_2.0_a639b : Constant  Value=2.0
  Constant_2.0_e12b9 : Constant  Value=2.0
  Constant_D_6c81a : Constant  Value=D
  Constant_H_89195 : Constant  Value=H
  Constant_f0_836c5 : Constant  Value=f0
  Constant_f0_9d3e3 : Constant  Value=f0
  Constant_f0_ba1be : Constant  Value=f0
  Constant_pi_477bc : Constant  Value=pi
  Constant_pi_9608b : Constant  Value=pi
  Constant_pi_b1771 : Constant  Value=pi
  Constant_x_dd_64921 : Constant  Value=x_dd
  Constant_x_dd_b8434 : Constant  Value=x_dd
  Constant_x_dd_fc1ac : Constant  Value=x_dd
  Constant_x_ddd_1db81 : Constant  Value=x_ddd
  Constant_x_ddd_3ab91 : Constant  Value=x_ddd
  Constant_x_ddd_afffa : Constant  Value=x_ddd
  Constant_x_l_05418 : Constant  Value=x_l
  Constant_x_l_4f13b : Constant  Value=x_l
  Constant_x_l_a3c43 : Constant  Value=x_l
  Constant_x_l_d4cbb : Constant  Value=x_l
  Constant_x_l_e2469 : Constant  Value=x_l
  Constant_x_l_f3daa : Constant  Value=x_l
  Constant_x_qd_2f788 : Constant  Value=x_qd
  Constant_x_qd_ab56a : Constant  Value=x_qd
  Constant_x_qd_afff6 : Constant  Value=x_qd
  Constant_x_qdd_3c9a2 : Constant  Value=x_qdd
  Constant_x_qdd_a02a9 : Constant  Value=x_qdd
  Constant_x_qdd_f1cfc : Constant  Value=x_qdd
  Divide_02fc4 : Product  Inputs=*/
  Divide_14b8b : Product  Inputs=*/
  Divide_1e7ee : Product  Inputs=*/
  Divide_223d5 : Product  Inputs=*/
  Divide_cca63 : Product  Inputs=*/
  Divide_fc5f6 : Product  Inputs=*/
  Divide_fdd42 : Product  Inputs=*/
  Product_10baf : Product
  Product_2a668 : Product
  Product_2fd84 : Product
  Product_45d97 : Product
  Product_5432a : Product
  Product_68041 : Product
  Product_6bf34 : Product
  Product_6c6fb : Product
  Product_78b21 : Product
  Product_80b89 : Product
  Product_81dd7 : Product
  Product_8b27f : Product
  Product_8fc9c : Product
  Product_9874c : Product
  Product_989a1 : Product
  Product_b7127 : Product
  Product_be021 : Product
  Product_d5640 : Product
  Product_dddc3 : Product
  Product_e2292 : Product
  Product_e6880 : Product
  Product_f1028 : Product
  Subtract_10067 : Sum  Inputs=+-
  Subtract_3dbff : Sum  Inputs=+-
  Subtract_42270 : Sum  Inputs=+-
  Subtract_4ca15 : Sum  Inputs=+-
  Subtract_5d209 : Sum  Inputs=+-
  Subtract_8910e : Sum  Inputs=+-
  Subtract_cee62 : Sum  Inputs=+-
  Subtract_f3870 : Sum  Inputs=+-
  Blockout_d_w_SG_D_3_cf3fb : Outport
  wires:
  Constant_x_qd_afff6/1 -> Subtract_8910e/1
  Subtract_3dbff/1 -> Product_e2292/2
  Subtract_10067/1 -> Divide_cca63/1
  Constant_-1_a5909/1 -> Product_9874c/1
  Add_d2f95/1 -> Product_81dd7/2
  Constant_x_qdd_f1cfc/1 -> Subtract_8910e/2
  Subtract_cee62/1 -> Product_10baf/2
  Constant_x_l_a3c43/1 -> Product_9874c/2
  State_psi_d_SG_D_3_9af62/1 -> Add_942e8/2
  Add_883c3/1 -> Divide_14b8b/2
  Constant_x_dd_b8434/1 -> Subtract_f3870/1
  Constant_x_l_e2469/1 -> Product_6c6fb/2
  Constant_-1_86e24/1 -> Product_6bf34/1
  Divide_fc5f6/1 -> Subtract_42270/2
  Constant_x_ddd_afffa/1 -> Subtract_3dbff/2
  Constant_x_qdd_3c9a2/1 -> Add_d2f95/2
  Constant_pi_9608b/1 -> Product_45d97/2
  Product_9874c/1 -> Add_d2f95/1
  Constant_-2.0_47383/1 -> Product_989a1/1
  Constant_-1_64dcd/1 -> Product_6c6fb/1
  Constant_2.0_a639b/1 -> Product_b7127/1
  Product_989a1/1 -> Product_5432a/1
  Constant_-1_233d8/1 -> Product_8b27f/1
  Subtract_5d209/1 -> Add_2a10b/1
  Constant_x_l_f3daa/1 -> Product_8b27f/2
  Constant_x_l_d4cbb/1 -> Subtract_cee62/2
  Constant_-1_3c74a/1 -> Product_8fc9c/1
  State_psi_1d_SG_D_3_df021/1 -> Product_8fc9c/2
  Constant_x_dd_64921/1 -> Subtract_3dbff/1
  Product_8fc9c/1 -> Product_e2292/1
  State_psi_gq_SG_D_3_617ad/1 -> Product_81dd7/1
  Constant_x_qd_2f788/1 -> Add_883c3/2
  Product_6c6fb/1 -> Add_883c3/1
  State_psi_kq_SG_D_3_92701/1 -> Product_be021/1
  Subtract_8910e/1 -> Product_be021/2
  Product_b7127/1 -> Product_68041/1
  Product_5432a/1 -> Add_bd96e/1
  Product_8b27f/1 -> Add_d4927/1
  State_psi_q_SG_D_3_f932d/1 -> Product_d5640/1
  Constant_x_qd_ab56a/1 -> Add_d4927/2
  Constant_x_l_4f13b/1 -> Subtract_f3870/2
  Constant_x_ddd_1db81/1 -> Subtract_cee62/1
  Constant_x_l_05418/1 -> Subtract_4ca15/2
  Product_81dd7/1 -> Divide_14b8b/1
  Product_be021/1 -> Divide_223d5/1
  Add_d4927/1 -> Divide_223d5/2
  Product_e2292/1 -> Divide_1e7ee/1
  Subtract_f3870/1 -> Divide_1e7ee/2
  Constant_2.0_3f110/1 -> Product_45d97/1
  State_psi_fd_SG_D_3_b5ce7/1 -> Product_10baf/1
  Constant_x_dd_fc1ac/1 -> Subtract_4ca15/1
  Divide_14b8b/1 -> Subtract_5d209/1
  Product_10baf/1 -> Divide_fc5f6/1
  Divide_223d5/1 -> Subtract_5d209/2
  Divide_1e7ee/1 -> Add_942e8/1
  Product_e6880/1 -> Subtract_10067/2
  Subtract_4ca15/1 -> Divide_fc5f6/2
  Constant_pi_b1771/1 -> Product_989a1/2
  Constant_pi_477bc/1 -> Product_b7127/2
  Constant_-1_12918/1 -> Product_80b89/1
  State_psi_d_SG_D_3_b825f/1 -> Product_80b89/2
  State_psi_q_SG_D_3_c3d2e/1 -> Add_2a10b/2
  Add_942e8/1 -> Subtract_42270/1
  Constant_f0_9d3e3/1 -> Product_5432a/2
  Product_80b89/1 -> Product_f1028/1
  Add_2a10b/1 -> Product_f1028/2
  Subtract_42270/1 -> Product_d5640/2
  Constant_D_6c81a/1 -> Product_6bf34/2
  State_w_SG_D_3_c3b06/1 -> Add_bd96e/2
  Product_45d97/1 -> Product_2a668/1
  State_T_m_SG_D_3_e3476/1 -> Product_2a668/2
  Product_f1028/1 -> Divide_02fc4/1
  Constant_x_qdd_a02a9/1 -> Divide_02fc4/2
  Product_d5640/1 -> Divide_fdd42/1
  Constant_x_ddd_3ab91/1 -> Divide_fdd42/2
  Product_6bf34/1 -> Product_78b21/1
  Add_bd96e/1 -> Product_78b21/2
  Product_2a668/1 -> Product_2fd84/1
  Constant_f0_836c5/1 -> Product_2fd84/2
  Constant_f0_ba1be/1 -> Product_68041/2
  Divide_02fc4/1 -> Add_d3e9c/1
  Divide_fdd42/1 -> Add_d3e9c/2
  Product_78b21/1 -> Add_9e5f9/1
  Product_2fd84/1 -> Add_9e5f9/2
  Product_68041/1 -> Product_e6880/1
  Add_d3e9c/1 -> Product_e6880/2
  Add_9e5f9/1 -> Subtract_10067/1
  Constant_2.0_e12b9/1 -> Product_dddc3/1
  Constant_H_89195/1 -> Product_dddc3/2
  Product_dddc3/1 -> Divide_cca63/2
  Divide_cca63/1 -> Blockout_d_w_SG_D_3_cf3fb/1

== system case5/SG_D_3/i_d_SG_D_3_block ==
  note: i_d_SG_D_3 in case5
      | $\frac{\sin\left(\theta _{\mathrm{SG},D,3}\right)\,\left(\frac{\psi _{\mathrm{1d},\mathrm{SG},D,3}\,\left(x_{\mathrm{dd}}-x_{\mathrm{ddd}}\right)}{x_{\mathrm{dd}}-x_{l}}-\psi _{d,\mathrm{SG},D,3}+\frac{\psi _{\mathrm{fd},\mathrm{SG},D,3}\,\left(x_{\mathrm{ddd}}-x_{l}\right)}{x_{\mathrm{dd}}-x_{l}}\right)}{x_{\mathrm{ddd}}}-\frac{\cos\left(\theta _{\mathrm{SG},D,3}\right)\,\left(\psi _{q,\mathrm{SG},D,3}+\frac{\psi _{\mathrm{gq},\mathrm{SG},D,3}\,\left(x_{l}-x_{\mathrm{qdd}}\right)}{x_{l}-x_{\mathrm{qd}}}+\frac{\psi _{\mathrm{kq},\mathrm{SG},D,3}\,\left(x_{\mathrm{qd}}-x_{\mathrm{qdd}}\right)}{x_{l}-x_{\mathrm{qd}}}\right)}{x_{\mathrm{qdd}}}$
      | Automatically generated on 2025-10-31 19:13:16 .
  State_psi_gq_SG_D_3_83e92 : Inport
  State_psi_kq_SG_D_3_2d375 : Inport  Port=2
  State_psi_q_SG_D_3_70eb0 : Inport  Port=3
  State_theta_SG_D_3_03d7d : Inport  Port=4
  State_psi_1d_SG_D_3_ba81f : Inport  Port=5
  State_psi_d_SG_D_3_22276 : Inport  Port=6
  State_psi_fd_SG_D_3_ca9c0 : Inport  Port=7
  State_theta_SG_D_3_5a6b6 : Inport  Port=8
  Add_0d683 : Sum
  Add_38002 : Sum
  Add_93b38 : Sum
  Add_ba822 : Sum
  Add_d2f2f : Sum
  Constant_-1_0b865 : Constant  Value=-1
  Constant_-1_1462c : Constant  Value=-1
  Constant_-1_97742 : Constant  Value=-1
  Constant_-1_b84aa : Constant  Value=-1
  Constant_-1_c2366 : Constant  Value=-1
  Constant_x_dd_629c7 : Constant  Value=x_dd
  Constant_x_dd_83ce3 : Constant  Value=x_dd
  Constant_x_dd_973d1 : Constant  Value=x_dd
  Constant_x_ddd_08114 : Constant  Value=x_ddd
  Constant_x_ddd_6a71a : Constant  Value=x_ddd
  Constant_x_ddd_f8dac : Constant  Value=x_ddd
  Constant_x_l_328f1 : Constant  Value=x_l
  Constant_x_l_538f7 : Constant  Value=x_l
  Constant_x_l_7aeae : Constant  Value=x_l
  Constant_x_l_82ec0 : Constant  Value=x_l
  Constant_x_l_a7d89 : Constant  Value=x_l
  Constant_x_l_aca8c : Constant  Value=x_l
  Constant_x_qd_051a2 : Constant  Value=x_qd
  Constant_x_qd_3943d : Constant  Value=x_qd
  Constant_x_qd_4b75a : Constant  Value=x_qd
  Constant_x_qdd_2e248 : Constant  Value=x_qdd
  Constant_x_qdd_74c3e : Constant  Value=x_qdd
  Constant_x_qdd_ac47a : Constant  Value=x_qdd
  Divide_10da7 : Product  Inputs=*/
  Divide_2a074 : Product  Inputs=*/
  Divide_2be65 : Product  Inputs=*/
  Divide_6c36b : Product  Inputs=*/
  Divide_6d94c : Product  Inputs=*/
  Divide_c67aa : Product  Inputs=*/
  MathFunc_cos_f4efa : Trigonometry  Operator=cos
  MathFunc_sin_1eacb : Trigonometry
  Product_1d96f : Product
  Product_23356 : Product
  Product_3a179 : Product
  Product_586d7 : Product
  Product_5e41d : Product
  Product_6f4a6 : Product
  Product_9bea4 : Product
  Product_ce93a : Product
  Product_e75b2 : Product
  Product_e8c19 : Product
  Product_fd097 : Product
  Subtract_09adc : Sum  Inputs=+-
  Subtract_38ca6 : Sum  Inputs=+-
  Subtract_71202 : Sum  Inputs=+-
  Subtract_7f130 : Sum  Inputs=+-
  Subtract_87991 : Sum  Inputs=+-
  Subtract_98d1e : Sum  Inputs=+-
  Subtract_a641a : Sum  Inputs=+-
  Subtract_ba879 : Sum  Inputs=+-
  Blockout_i_d_SG_D_3_8b105 : Outport
  wires:
  Constant_x_qd_4b75a/1 -> Subtract_38ca6/1
  Subtract_98d1e/1 -> Blockout_i_d_SG_D_3_8b105/1
  Constant_-1_1462c/1 -> Product_fd097/1
  Constant_x_l_538f7/1 -> Product_e8c19/2
  Constant_x_qdd_2e248/1 -> Add_ba822/2
  Constant_x_qdd_74c3e/1 -> Subtract_38ca6/2
  Constant_x_l_a7d89/1 -> Product_fd097/2
  Divide_2a074/1 -> Subtract_98d1e/1
  Product_fd097/1 -> Add_ba822/1
  Constant_x_ddd_6a71a/1 -> Subtract_87991/2
  Constant_-1_97742/1 -> Product_e8c19/1
  Constant_-1_0b865/1 -> Product_6f4a6/1
  Constant_x_l_328f1/1 -> Product_6f4a6/2
  State_psi_1d_SG_D_3_ba81f/1 -> Product_e75b2/2
  State_psi_gq_SG_D_3_83e92/1 -> Product_ce93a/1
  Product_e75b2/1 -> Product_3a179/1
  Add_ba822/1 -> Product_ce93a/2
  Product_e8c19/1 -> Add_0d683/1
  Constant_x_qd_051a2/1 -> Add_0d683/2
  State_psi_kq_SG_D_3_2d375/1 -> Product_5e41d/1
  Subtract_7f130/1 -> Divide_10da7/2
  Subtract_38ca6/1 -> Product_5e41d/2
  Product_6f4a6/1 -> Add_d2f2f/1
  Constant_x_ddd_f8dac/1 -> Subtract_71202/1
  Constant_x_qd_3943d/1 -> Add_d2f2f/2
  Constant_-1_b84aa/1 -> Product_e75b2/1
  Constant_x_dd_83ce3/1 -> Subtract_87991/1
  Product_ce93a/1 -> Divide_c67aa/1
  Add_0d683/1 -> Divide_c67aa/2
  Product_5e41d/1 -> Divide_2be65/1
  Add_d2f2f/1 -> Divide_2be65/2
  Divide_10da7/1 -> Subtract_09adc/2
  Subtract_87991/1 -> Product_3a179/2
  State_theta_SG_D_3_03d7d/1 -> MathFunc_cos_f4efa/1
  Constant_x_dd_973d1/1 -> Subtract_a641a/1
  Product_23356/1 -> Product_9bea4/1
  Constant_x_l_82ec0/1 -> Subtract_a641a/2
  Add_38002/1 -> Subtract_09adc/1
  Constant_x_l_7aeae/1 -> Subtract_71202/2
  State_theta_SG_D_3_5a6b6/1 -> MathFunc_sin_1eacb/1
  Divide_c67aa/1 -> Subtract_ba879/1
  Add_93b38/1 -> Product_23356/2
  Divide_2be65/1 -> Subtract_ba879/2
  Product_3a179/1 -> Divide_6d94c/1
  Subtract_a641a/1 -> Divide_6d94c/2
  State_psi_fd_SG_D_3_ca9c0/1 -> Product_586d7/1
  Divide_6c36b/1 -> Subtract_98d1e/2
  Subtract_71202/1 -> Product_586d7/2
  Constant_x_dd_629c7/1 -> Subtract_7f130/1
  Subtract_ba879/1 -> Add_93b38/1
  Constant_x_l_aca8c/1 -> Subtract_7f130/2
  Constant_-1_c2366/1 -> Product_23356/1
  State_psi_q_SG_D_3_70eb0/1 -> Add_93b38/2
  Divide_6d94c/1 -> Add_38002/1
  State_psi_d_SG_D_3_22276/1 -> Add_38002/2
  Product_586d7/1 -> Divide_10da7/1
  MathFunc_cos_f4efa/1 -> Product_9bea4/2
  MathFunc_sin_1eacb/1 -> Product_1d96f/2
  Subtract_09adc/1 -> Product_1d96f/1
  Product_9bea4/1 -> Divide_2a074/1
  Constant_x_qdd_ac47a/1 -> Divide_2a074/2
  Product_1d96f/1 -> Divide_6c36b/1
  Constant_x_ddd_08114/1 -> Divide_6c36b/2
